simulink model "gm_I2S"  (R2023b)
settings: Solver=VariableStepAuto  StartTime=0.0  StopTime=10000  RelTol=1e-3
undefined symbols (not defined in the file or in its folder): cnt1_LRCLK, cnt2_SCLK, SH_R
libraries: hdlsllib x10
(part 5 of 5)

== system gm_I2S/I2S/PISO_SHIFT_REG_RIGHT1/Subsystem/MUX22 ==
  note: SEL=0 ==> IN1
  In1 : Inport
  In2 : Inport  Port=2
  SEL : Inport  Port=3  OutDataTypeStr=boolean
  Logical Operator : Logic  AllPortsSameDT=off  OutDataTypeStr=boolean
  Logical Operator1 : Logic  AllPortsSameDT=off  OutDataTypeStr=boolean
  Logical Operator2 : Logic  Operator=OR  AllPortsSameDT=off  OutDataTypeStr=boolean
  Logical Operator3 : Logic  Operator=NOT  AllPortsSameDT=off  OutDataTypeStr=boolean
  Out1 : Outport  VectorParamsAs1DForOutWhenUnconnected=off
  wires:
  In2/1 -> Logical Operator1/2
  Logical Operator2/1 -> Out1/1
  Logical Operator/1 -> Logical Operator2/1
  Logical Operator1/1 -> Logical Operator2/2
  Logical Operator3/1 -> Logical Operator/2
  SEL/1 -> Logical Operator1/1, Logical Operator3/1
  In1/1 -> Logical Operator/1

== system gm_I2S/I2S/PISO_SHIFT_REG_RIGHT1/Subsystem/MUX23 ==
  note: SEL=0 ==> IN1
  In1 : Inport
  In2 : Inport  Port=2
  SEL : Inport  Port=3  OutDataTypeStr=boolean
  Logical Operator : Logic  AllPortsSameDT=off  OutDataTypeStr=boolean
  Logical Operator1 : Logic  AllPortsSameDT=off  OutDataTypeStr=boolean
  Logical Operator2 : Logic  Operator=OR  AllPortsSameDT=off  OutDataTypeStr=boolean
  Logical Operator3 : Logic  Operator=NOT  AllPortsSameDT=off  OutDataTypeStr=boolean
  Out1 : Outport  VectorParamsAs1DForOutWhenUnconnected=off
  wires:
  In2/1 -> Logical Operator1/2
  Logical Operator2/1 -> Out1/1
  Logical Operator/1 -> Logical Operator2/1
  Logical Operator1/1 -> Logical Operator2/2
  Logical Operator3/1 -> Logical Operator/2
  SEL/1 -> Logical Operator1/1, Logical Operator3/1
  In1/1 -> Logical Operator/1

== system gm_I2S/I2S/PISO_SHIFT_REG_RIGHT1/Subsystem/MUX24 ==
  note: SEL=0 ==> IN1
  In1 : Inport
  In2 : Inport  Port=2
  SEL : Inport  Port=3  OutDataTypeStr=boolean
  Logical Operator : Logic  AllPortsSameDT=off  OutDataTypeStr=boolean
  Logical Operator1 : Logic  AllPortsSameDT=off  OutDataTypeStr=boolean
  Logical Operator2 : Logic  Operator=OR  AllPortsSameDT=off  OutDataTypeStr=boolean
  Logical Operator3 : Logic  Operator=NOT  AllPortsSameDT=off  OutDataTypeStr=boolean
  Out1 : Outport  VectorParamsAs1DForOutWhenUnconnected=off
  wires:
  In2/1 -> Logical Operator1/2
  Logical Operator2/1 -> Out1/1
  Logical Operator/1 -> Logical Operator2/1
  Logical Operator1/1 -> Logical Operator2/2
  Logical Operator3/1 -> Logical Operator/2
  SEL/1 -> Logical Operator1/1, Logical Operator3/1
  In1/1 -> Logical Operator/1

== system gm_I2S/I2S/PISO_SHIFT_REG_RIGHT1/Subsystem/MUX25 ==
  note: SEL=0 ==> IN1
  In1 : Inport
  In2 : Inport  Port=2
  SEL : Inport  Port=3  OutDataTypeStr=boolean
  Logical Operator : Logic  AllPortsSameDT=off  OutDataTypeStr=boolean
  Logical Operator1 : Logic  AllPortsSameDT=off  OutDataTypeStr=boolean
  Logical Operator2 : Logic  Operator=OR  AllPortsSameDT=off  OutDataTypeStr=boolean
  Logical Operator3 : Logic  Operator=NOT  AllPortsSameDT=off  OutDataTypeStr=boolean
  Out1 : Outport  VectorParamsAs1DForOutWhenUnconnected=off
  wires:
  In2/1 -> Logical Operator1/2
  Logical Operator2/1 -> Out1/1
  Logical Operator/1 -> Logical Operator2/1
  Logical Operator1/1 -> Logical Operator2/2
  Logical Operator3/1 -> Logical Operator/2
  SEL/1 -> Logical Operator1/1, Logical Operator3/1
  In1/1 -> Logical Operator/1

== system gm_I2S/I2S/PISO_SHIFT_REG_RIGHT1/Subsystem/MUX26 ==
  note: SEL=0 ==> IN1
  In1 : Inport
  In2 : Inport  Port=2
  SEL : Inport  Port=3  OutDataTypeStr=boolean
  Logical Operator : Logic  AllPortsSameDT=off  OutDataTypeStr=boolean
  Logical Operator1 : Logic  AllPortsSameDT=off  OutDataTypeStr=boolean
  Logical Operator2 : Logic  Operator=OR  AllPortsSameDT=off  OutDataTypeStr=boolean
  Logical Operator3 : Logic  Operator=NOT  AllPortsSameDT=off  OutDataTypeStr=boolean
  Out1 : Outport  VectorParamsAs1DForOutWhenUnconnected=off
  wires:
  In2/1 -> Logical Operator1/2
  Logical Operator2/1 -> Out1/1
  Logical Operator/1 -> Logical Operator2/1
  Logical Operator1/1 -> Logical Operator2/2
  Logical Operator3/1 -> Logical Operator/2
  SEL/1 -> Logical Operator1/1, Logical Operator3/1
  In1/1 -> Logical Operator/1

== system gm_I2S/I2S/PISO_SHIFT_REG_RIGHT1/Subsystem/MUX27 ==
  note: SEL=0 ==> IN1
  In1 : Inport
  In2 : Inport  Port=2
  SEL : Inport  Port=3  OutDataTypeStr=boolean
  Logical Operator : Logic  AllPortsSameDT=off  OutDataTypeStr=boolean
  Logical Operator1 : Logic  AllPortsSameDT=off  OutDataTypeStr=boolean
  Logical Operator2 : Logic  Operator=OR  AllPortsSameDT=off  OutDataTypeStr=boolean
  Logical Operator3 : Logic  Operator=NOT  AllPortsSameDT=off  OutDataTypeStr=boolean
  Out1 : Outport  VectorParamsAs1DForOutWhenUnconnected=off
  wires:
  In2/1 -> Logical Operator1/2
  Logical Operator2/1 -> Out1/1
  Logical Operator/1 -> Logical Operator2/1
  Logical Operator1/1 -> Logical Operator2/2
  Logical Operator3/1 -> Logical Operator/2
  SEL/1 -> Logical Operator1/1, Logical Operator3/1
  In1/1 -> Logical Operator/1

== system gm_I2S/I2S/PISO_SHIFT_REG_RIGHT1/Subsystem/MUX28 ==
  note: SEL=0 ==> IN1
  In1 : Inport
  In2 : Inport  Port=2
  SEL : Inport  Port=3  OutDataTypeStr=boolean
  Logical Operator : Logic  AllPortsSameDT=off  OutDataTypeStr=boolean
  Logical Operator1 : Logic  AllPortsSameDT=off  OutDataTypeStr=boolean
  Logical Operator2 : Logic  Operator=OR  AllPortsSameDT=off  OutDataTypeStr=boolean
  Logical Operator3 : Logic  Operator=NOT  AllPortsSameDT=off  OutDataTypeStr=boolean
  Out1 : Outport  VectorParamsAs1DForOutWhenUnconnected=off
  wires:
  In2/1 -> Logical Operator1/2
  Logical Operator2/1 -> Out1/1
  Logical Operator/1 -> Logical Operator2/1
  Logical Operator1/1 -> Logical Operator2/2
  Logical Operator3/1 -> Logical Operator/2
  SEL/1 -> Logical Operator1/1, Logical Operator3/1
  In1/1 -> Logical Operator/1

== system gm_I2S/I2S/PISO_SHIFT_REG_RIGHT1/Subsystem/MUX29 ==
  note: SEL=0 ==> IN1
  In1 : Inport
  In2 : Inport  Port=2
  SEL : Inport  Port=3  OutDataTypeStr=boolean
  Logical Operator : Logic  AllPortsSameDT=off  OutDataTypeStr=boolean
  Logical Operator1 : Logic  AllPortsSameDT=off  OutDataTypeStr=boolean
  Logical Operator2 : Logic  Operator=OR  AllPortsSameDT=off  OutDataTypeStr=boolean
  Logical Operator3 : Logic  Operator=NOT  AllPortsSameDT=off  OutDataTypeStr=boolean
  Out1 : Outport  VectorParamsAs1DForOutWhenUnconnected=off
  wires:
  In2/1 -> Logical Operator1/2
  Logical Operator2/1 -> Out1/1
  Logical Operator/1 -> Logical Operator2/1
  Logical Operator1/1 -> Logical Operator2/2
  Logical Operator3/1 -> Logical Operator/2
  SEL/1 -> Logical Operator1/1, Logical Operator3/1
  In1/1 -> Logical Operator/1

== system gm_I2S/I2S/PISO_SHIFT_REG_RIGHT1/Subsystem/MUX3 ==
  note: SEL=0 ==> IN1
  In1 : Inport
  In2 : Inport  Port=2
  SEL : Inport  Port=3  OutDataTypeStr=boolean
  Logical Operator : Logic  AllPortsSameDT=off  OutDataTypeStr=boolean
  Logical Operator1 : Logic  AllPortsSameDT=off  OutDataTypeStr=boolean
  Logical Operator2 : Logic  Operator=OR  AllPortsSameDT=off  OutDataTypeStr=boolean
  Logical Operator3 : Logic  Operator=NOT  AllPortsSameDT=off  OutDataTypeStr=boolean
  Out1 : Outport  VectorParamsAs1DForOutWhenUnconnected=off
  wires:
  In2/1 -> Logical Operator1/2
  Logical Operator2/1 -> Out1/1
  Logical Operator/1 -> Logical Operator2/1
  Logical Operator1/1 -> Logical Operator2/2
  Logical Operator3/1 -> Logical Operator/2
  SEL/1 -> Logical Operator1/1, Logical Operator3/1
  In1/1 -> Logical Operator/1

== system gm_I2S/I2S/PISO_SHIFT_REG_RIGHT1/Subsystem/MUX30 ==
  note: SEL=0 ==> IN1
  In1 : Inport
  In2 : Inport  Port=2
  SEL : Inport  Port=3  OutDataTypeStr=boolean
  Logical Operator : Logic  AllPortsSameDT=off  OutDataTypeStr=boolean
  Logical Operator1 : Logic  AllPortsSameDT=off  OutDataTypeStr=boolean
  Logical Operator2 : Logic  Operator=OR  AllPortsSameDT=off  OutDataTypeStr=boolean
  Logical Operator3 : Logic  Operator=NOT  AllPortsSameDT=off  OutDataTypeStr=boolean
  Out1 : Outport  VectorParamsAs1DForOutWhenUnconnected=off
  wires:
  In2/1 -> Logical Operator1/2
  Logical Operator2/1 -> Out1/1
  Logical Operator/1 -> Logical Operator2/1
  Logical Operator1/1 -> Logical Operator2/2
  Logical Operator3/1 -> Logical Operator/2
  SEL/1 -> Logical Operator1/1, Logical Operator3/1
  In1/1 -> Logical Operator/1

== system gm_I2S/I2S/PISO_SHIFT_REG_RIGHT1/Subsystem/MUX31 ==
  note: SEL=0 ==> IN1
  In1 : Inport
  In2 : Inport  Port=2
  SEL : Inport  Port=3  OutDataTypeStr=boolean
  Logical Operator : Logic  AllPortsSameDT=off  OutDataTypeStr=boolean
  Logical Operator1 : Logic  AllPortsSameDT=off  OutDataTypeStr=boolean
  Logical Operator2 : Logic  Operator=OR  AllPortsSameDT=off  OutDataTypeStr=boolean
  Logical Operator3 : Logic  Operator=NOT  AllPortsSameDT=off  OutDataTypeStr=boolean
  Out1 : Outport  VectorParamsAs1DForOutWhenUnconnected=off
  wires:
  In2/1 -> Logical Operator1/2
  Logical Operator2/1 -> Out1/1
  Logical Operator/1 -> Logical Operator2/1
  Logical Operator1/1 -> Logical Operator2/2
  Logical Operator3/1 -> Logical Operator/2
  SEL/1 -> Logical Operator1/1, Logical Operator3/1
  In1/1 -> Logical Operator/1

== system gm_I2S/I2S/PISO_SHIFT_REG_RIGHT1/Subsystem/MUX4 ==
  note: SEL=0 ==> IN1
  In1 : Inport
  In2 : Inport  Port=2
  SEL : Inport  Port=3  OutDataTypeStr=boolean
  Logical Operator : Logic  AllPortsSameDT=off  OutDataTypeStr=boolean
  Logical Operator1 : Logic  AllPortsSameDT=off  OutDataTypeStr=boolean
  Logical Operator2 : Logic  Operator=OR  AllPortsSameDT=off  OutDataTypeStr=boolean
  Logical Operator3 : Logic  Operator=NOT  AllPortsSameDT=off  OutDataTypeStr=boolean
  Out1 : Outport  VectorParamsAs1DForOutWhenUnconnected=off
  wires:
  In2/1 -> Logical Operator1/2
  Logical Operator2/1 -> Out1/1
  Logical Operator/1 -> Logical Operator2/1
  Logical Operator1/1 -> Logical Operator2/2
  Logical Operator3/1 -> Logical Operator/2
  SEL/1 -> Logical Operator1/1, Logical Operator3/1
  In1/1 -> Logical Operator/1

== system gm_I2S/I2S/PISO_SHIFT_REG_RIGHT1/Subsystem/MUX5 ==
  note: SEL=0 ==> IN1
  In1 : Inport
  In2 : Inport  Port=2
  SEL : Inport  Port=3  OutDataTypeStr=boolean
  Logical Operator : Logic  AllPortsSameDT=off  OutDataTypeStr=boolean
  Logical Operator1 : Logic  AllPortsSameDT=off  OutDataTypeStr=boolean
  Logical Operator2 : Logic  Operator=OR  AllPortsSameDT=off  OutDataTypeStr=boolean
  Logical Operator3 : Logic  Operator=NOT  AllPortsSameDT=off  OutDataTypeStr=boolean
  Out1 : Outport  VectorParamsAs1DForOutWhenUnconnected=off
  wires:
  In2/1 -> Logical Operator1/2
  Logical Operator2/1 -> Out1/1
  Logical Operator/1 -> Logical Operator2/1
  Logical Operator1/1 -> Logical Operator2/2
  Logical Operator3/1 -> Logical Operator/2
  SEL/1 -> Logical Operator1/1, Logical Operator3/1
  In1/1 -> Logical Operator/1

== system gm_I2S/I2S/PISO_SHIFT_REG_RIGHT1/Subsystem/MUX6 ==
  note: SEL=0 ==> IN1
  In1 : Inport
  In2 : Inport  Port=2
  SEL : Inport  Port=3  OutDataTypeStr=boolean
  Logical Operator : Logic  AllPortsSameDT=off  OutDataTypeStr=boolean
  Logical Operator1 : Logic  AllPortsSameDT=off  OutDataTypeStr=boolean
  Logical Operator2 : Logic  Operator=OR  AllPortsSameDT=off  OutDataTypeStr=boolean
  Logical Operator3 : Logic  Operator=NOT  AllPortsSameDT=off  OutDataTypeStr=boolean
  Out1 : Outport  VectorParamsAs1DForOutWhenUnconnected=off
  wires:
  In2/1 -> Logical Operator1/2
  Logical Operator2/1 -> Out1/1
  Logical Operator/1 -> Logical Operator2/1
  Logical Operator1/1 -> Logical Operator2/2
  Logical Operator3/1 -> Logical Operator/2
  SEL/1 -> Logical Operator1/1, Logical Operator3/1
  In1/1 -> Logical Operator/1

== system gm_I2S/I2S/PISO_SHIFT_REG_RIGHT1/Subsystem/MUX7 ==
  note: SEL=0 ==> IN1
  In1 : Inport
  In2 : Inport  Port=2
  SEL : Inport  Port=3  OutDataTypeStr=boolean
  Logical Operator : Logic  AllPortsSameDT=off  OutDataTypeStr=boolean
  Logical Operator1 : Logic  AllPortsSameDT=off  OutDataTypeStr=boolean
  Logical Operator2 : Logic  Operator=OR  AllPortsSameDT=off  OutDataTypeStr=boolean
  Logical Operator3 : Logic  Operator=NOT  AllPortsSameDT=off  OutDataTypeStr=boolean
  Out1 : Outport  VectorParamsAs1DForOutWhenUnconnected=off
  wires:
  In2/1 -> Logical Operator1/2
  Logical Operator2/1 -> Out1/1
  Logical Operator/1 -> Logical Operator2/1
  Logical Operator1/1 -> Logical Operator2/2
  Logical Operator3/1 -> Logical Operator/2
  SEL/1 -> Logical Operator1/1, Logical Operator3/1
  In1/1 -> Logical Operator/1

== system gm_I2S/I2S/PISO_SHIFT_REG_RIGHT1/Subsystem/MUX8 ==
  note: SEL=0 ==> IN1
  In1 : Inport
  In2 : Inport  Port=2
  SEL : Inport  Port=3  OutDataTypeStr=boolean
  Logical Operator : Logic  AllPortsSameDT=off  OutDataTypeStr=boolean
  Logical Operator1 : Logic  AllPortsSameDT=off  OutDataTypeStr=boolean
  Logical Operator2 : Logic  Operator=OR  AllPortsSameDT=off  OutDataTypeStr=boolean
  Logical Operator3 : Logic  Operator=NOT  AllPortsSameDT=off  OutDataTypeStr=boolean
  Out1 : Outport  VectorParamsAs1DForOutWhenUnconnected=off
  wires:
  In2/1 -> Logical Operator1/2
  Logical Operator2/1 -> Out1/1
  Logical Operator/1 -> Logical Operator2/1
  Logical Operator1/1 -> Logical Operator2/2
  Logical Operator3/1 -> Logical Operator/2
  SEL/1 -> Logical Operator1/1, Logical Operator3/1
  In1/1 -> Logical Operator/1

== system gm_I2S/I2S/PISO_SHIFT_REG_RIGHT1/Subsystem/MUX9 ==
  note: SEL=0 ==> IN1
  In1 : Inport
  In2 : Inport  Port=2
  SEL : Inport  Port=3  OutDataTypeStr=boolean
  Logical Operator : Logic  AllPortsSameDT=off  OutDataTypeStr=boolean
  Logical Operator1 : Logic  AllPortsSameDT=off  OutDataTypeStr=boolean
  Logical Operator2 : Logic  Operator=OR  AllPortsSameDT=off  OutDataTypeStr=boolean
  Logical Operator3 : Logic  Operator=NOT  AllPortsSameDT=off  OutDataTypeStr=boolean
  Out1 : Outport  VectorParamsAs1DForOutWhenUnconnected=off
  wires:
  In2/1 -> Logical Operator1/2
  Logical Operator2/1 -> Out1/1
  Logical Operator/1 -> Logical Operator2/1
  Logical Operator1/1 -> Logical Operator2/2
  Logical Operator3/1 -> Logical Operator/2
  SEL/1 -> Logical Operator1/1, Logical Operator3/1
  In1/1 -> Logical Operator/1
